simulink model "s_ident1"  (Simulink 4.00)
settings: Solver=ode45  StartTime=0.0  StopTime=100  RelTol=1e-3
libraries: slident x1
settings Model: LastModifiedBy=Administrator  BlockReductionOpt=off

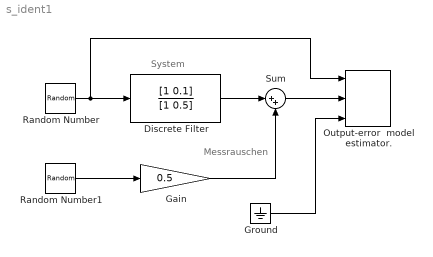
== system s_ident1 ==
  note: Messrauschen
  note: System
  Discrete Filter : DiscreteFilter  Numerator=[1 0.1]  Denominator=[1 0.5]  SampleTime=0.1  Realization=auto
  Gain : Gain  Gain=0.5  Multiplication=Element-wise(K.*u)  SaturateOnIntegerOverflow=on
  Ground : Ground
  Output-error  model estimator. : slident/Output-error  model estimator.  MaskParam1=256  MaskParam2=[2 1 0]  MaskParam3=64  MaskParam4=0.1
  Random Number : RandomNumber  Mean=0  Variance=1  Seed=0  SampleTime=0.1
  Random Number1 : RandomNumber  Mean=0  Variance=1  Seed=1479  SampleTime=0.1
  Sum : Sum  Inputs=|++  SaturateOnIntegerOverflow=on
  wires:
  Random Number/1 -> Discrete Filter/1, Output-error  model estimator./1
  Random Number1/1 -> Gain/1
  Discrete Filter/1 -> Sum/1
  Sum/1 -> Output-error  model estimator./2
  Gain/1 -> Sum/2
  Ground/1 -> Output-error  model estimator./3
